simulink model "Edr"  (R2020b)
settings: configuration reference "gen_config" (kept outside this file)
undefined symbols (not defined in the file): Edr_pwr_LossMap_AXIS, Edr_pwrInverterLosses_MAP, Edr_pwrMachineLosses_MAP, Edr_rpm_InvLossMap_AXIS, Edr_rpm_MachLossMap_AXIS, Edr_tq_MachLossMap_AXIS
settings Model: DataDictionary=Hybrid_vehicle.sldd  SimulationMode=accelerator  Creator=Georg  LastModifiedBy=jy
settings ConfigSetRef: SourceName=gen_config

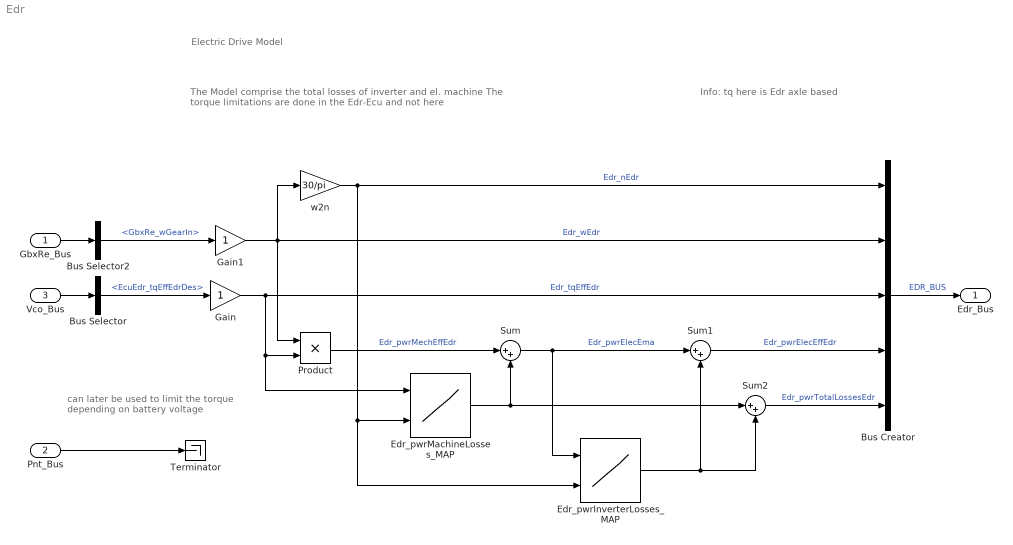
== system Edr ==
  note: Electric Drive Model
  note: Info:
      | tq here is Edr axle based
  note: The Model comprise the total losses of inverter and el. machine
      | The torque limitations are done in the Edr-Ecu and not here
  note: can later be used to limit the torque
      | depending on battery voltage
  GbxRe_Bus : Inport  OutDataTypeStr=Bus: GBXRE_BUS
  Pnt_Bus : Inport  Port=2  OutDataTypeStr=Bus: PNT_BUS
  Vco_Bus : Inport  Port=3  OutDataTypeStr=Bus: VCO_BUS
  Bus Creator : BusCreator  Inputs=5  OutDataTypeStr=Bus: EDR_BUS  NonVirtualBus=on
  Bus Selector : BusSelector  OutputSignals=EcuEdr_Bus.EcuEdr_tqEffEdrDes
  Bus Selector2 : BusSelector  OutputSignals=GbxRe_wGearIn
  Edr_pwrInverterLosses_MAP : Lookup_n-D  BreakpointsForDimension1=Edr_pwr_LossMap_AXIS  BreakpointsForDimension2=Edr_rpm_InvLossMap_AXIS  Table=Edr_pwrInverterLosses_MAP  ExtrapMethod=Clip  UseLastTableValue=on  InternalRulePriority=Speed  RndMeth=Simplest  InputSameDT=on
      settings: InputPortMap=u0,u1
  Edr_pwrMachineLosses_MAP : Lookup_n-D  BreakpointsForDimension1=Edr_tq_MachLossMap_AXIS  BreakpointsForDimension2=Edr_rpm_MachLossMap_AXIS  Table=Edr_pwrMachineLosses_MAP  ExtrapMethod=Clip  UseLastTableValue=on  InternalRulePriority=Speed  RndMeth=Simplest  InputSameDT=on
      settings: InputPortMap=u0,u1
  Gain : Gain
  Gain1 : Gain
  Product : Product
  Sum : Sum  Inputs=|++
  Sum1 : Sum  Inputs=|++
  Sum2 : Sum  Inputs=|++
  Terminator : Terminator
  w2n : Gain  Gain=30/pi
  Edr_Bus : Outport  OutDataTypeStr=Bus: EDR_BUS  VectorParamsAs1DForOutWhenUnconnected=off  BusOutputAsStruct=on
  wires:
  Gain/1 -> Edr_pwrMachineLosses_MAP/1, Product/2, Bus Creator/3  "Edr_tqEffEdr"
  Bus Selector2/1 -> Gain1/1  "<GbxRe_wGearIn>"
  GbxRe_Bus/1 -> Bus Selector2/1
  Bus Selector/1 -> Gain/1  "<EcuEdr_tqEffEdrDes>"
  Vco_Bus/1 -> Bus Selector/1
  Bus Creator/1 -> Edr_Bus/1  "EDR_BUS"
  Sum1/1 -> Bus Creator/4  "Edr_pwrElecEffEdr"
  Product/1 -> Sum/1  "Edr_pwrMechEffEdr"
  Pnt_Bus/1 -> Terminator/1
  Gain1/1 -> Bus Creator/2, w2n/1, Product/1  "Edr_wEdr"
  Edr_pwrInverterLosses_MAP/1 -> Sum1/2, Sum2/2
  w2n/1 -> Bus Creator/1, Edr_pwrInverterLosses_MAP/2, Edr_pwrMachineLosses_MAP/2  "Edr_nEdr"
  Sum/1 -> Sum1/1, Edr_pwrInverterLosses_MAP/1  "Edr_pwrElecEma"
  Sum2/1 -> Bus Creator/5  "Edr_pwrTotalLossesEdr"
  Edr_pwrMachineLosses_MAP/1 -> Sum/2, Sum2/1
